simulink subsystem "F3ph_to_F2ph"  (R2019b)
settings: Solver=VariableStepAuto  StartTime=0.0  StopTime=10.0  RelTol=1e-3
settings Model: Creator=Nathan Petersen  LastModifiedBy=Nathan Petersen

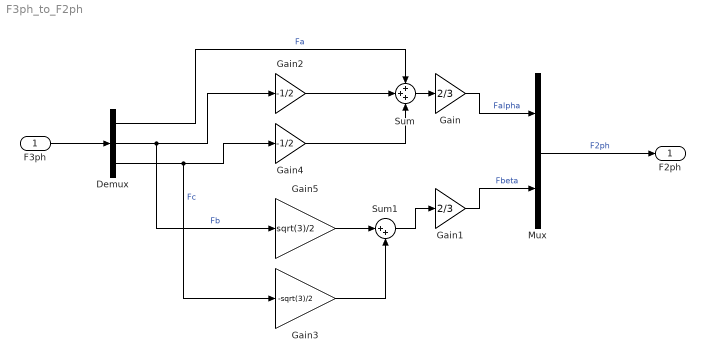
== system F3ph_to_F2ph ==
  F3ph : Inport  PortDimensions=3
  Demux : Demux  Outputs=3
  Gain : Gain  Gain=2/3
  Gain1 : Gain  Gain=2/3
  Gain2 : Gain  Gain=-1/2
  Gain3 : Gain  Gain=-sqrt(3)/2
  Gain4 : Gain  Gain=-1/2
  Gain5 : Gain  Gain=sqrt(3)/2
  Mux : Mux  Inputs=2
  Sum : Sum  Inputs=+++
  Sum1 : Sum  Inputs=|++
  F2ph : Outport  PortDimensions=2
  wires:
  Demux/2 -> Gain2/1, Gain5/1  "Fb"
  Gain/1 -> Mux/1  "Falpha"
  Gain4/1 -> Sum/3
  Gain1/1 -> Mux/2  "Fbeta"
  Sum1/1 -> Gain1/1
  Demux/3 -> Gain4/1, Gain3/1  "Fc"
  Gain3/1 -> Sum1/2
  Gain5/1 -> Sum1/1
  Sum/1 -> Gain/1
  Gain2/1 -> Sum/2
  Demux/1 -> Sum/1  "Fa"
  Mux/1 -> F2ph/1  "F2ph"
  F3ph/1 -> Demux/1
